simulink library "PECommon"  (Simulink 7.6)
settings: Solver=ode45  StartTime=0.0  StopTime=10.0  RelTol=1e-3
undefined symbols (not defined in the file or in its folder): DiscIntNeverNeededParam, Hydride, Metal, Nickel, Ts, Ts_Discrete
libraries: powerlib x24, simulink x14, PECommon x7, powerlib_extras x7, electricdrivelib x1, simulink_extras x1
(part 1 of 2)
settings Model: Creator=Hu Xaiolei  LastModifiedBy=Mike

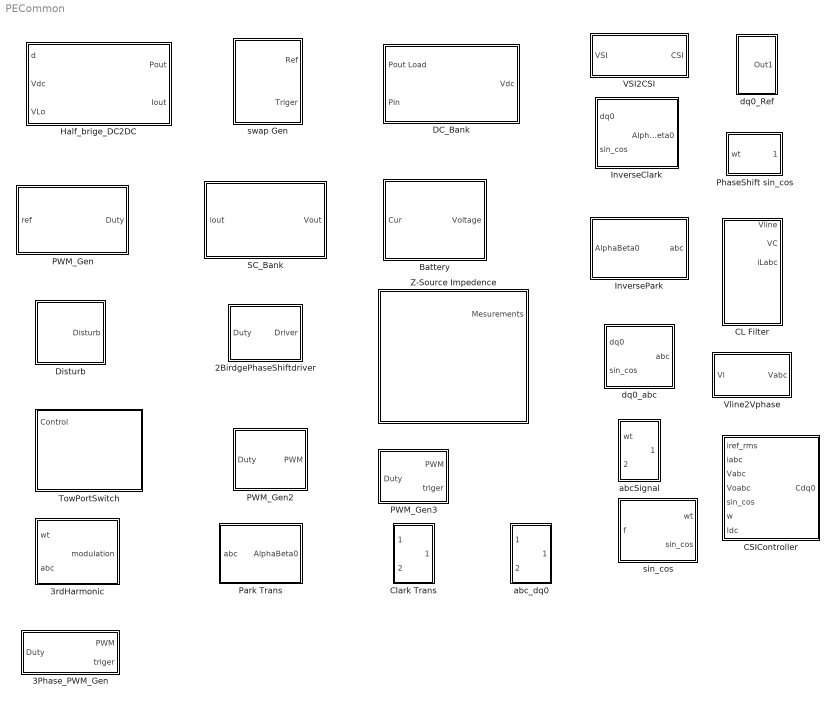
== system PECommon ==
  2BirdgePhaseShiftdriver : Subsystem  mask{fsps=10000}
      mask prompts: fsps "Freq of phase shift control"
      mask init:
      | TsPhaseShift = 1/fsps ;
      mask Display:
      | %plot([2 2 2 3 4 5 6 ],[3 5 5 3 3 5 5])
      | %plot([0 1 2 3 4 5 6 ], [0 0 2 2 0 0 2])
      | plot([0 1],[3 3])
      | plot([0 1],[0 0])
      | plot([1 1],[3 5])
      | plot([1 2],[5 5])
      | plot([1 2],[0 0])
      | plot([2 2],[0 2])
      | plot([2 3],[5 5])
      | plot([2 3],[2 2])
      | plot([3 3],[5 3])
      | plot([3 4],[3 3])
      | plot([3 4],[2 2])
      | plot([4 4],[2 0])
      | plot([4 5],[3 3])
      | plot([4 5],[0 0])
      | plot([5 5],[3 5])
      | plot([5 6],[5 5])
      | plot([5 6],[0 0])
      | plot([6 6],[0 2])
  3Phase_PWM_Gen : Subsystem  mask{Ts_Discrete=1e-6, f_tri=10e3, P_Delay=0}
      mask prompts: Ts_Discrete "Sample Time"; f_tri "Frequency of Sawtooth wave"; P_Delay "Phase Delay"
  3rdHarmonic : Subsystem  mask{SS=Original, ModeCtrl=0}
      mask prompts: SS "Source Selection"; ModeCtrl "Test"
      mask help:
      | 3 phase modulation
      | when Select original, the original A B C sine wave will be present
      | when select 3rd harmonic, 3rd harmonics will be added to A B C to increase
      | the utilization of DC bus.
      mask StyleString: popup(3rd Harmonic|Original),edit
      mask CallbackString:
      | if strcmp(get_param(gcb,'SS'),'Original')
      |     set_param(gcb,'ModeCtrl','0');
      | else
      |     set_param(gcb,'ModeCtrl','1');
      | end|
  Battery : Subsystem  mask{Value=200}
      mask prompts: Value "Battery Normal Voltage"
      mask Display:
      | image(imread('\pic\Battery_Service.jpg'))
      | port_label('input',1,'Current')
      | port_label('output',1,'Voltage')
  CL Filter : Subsystem  mask{L=1000e-6, C=100e-6, R=0.01}
      mask prompts: L "Inductance"; C "Capacitance"
  CSIController : Subsystem  mask{Kc=4.8000, Kp=6.9998, Ki=1.3333e+004, L=1000e-6, C=100e-6}
      mask prompts: Kc "inner loop gain"; Kp "Voltage loop gain"; Ki "Voltage loop integrator gain"; L "Inductance"; C "Capacitance"
  Clark Trans : Subsystem
  DC_Bank : Subsystem  mask{Cdc=0.47, Vdcinit=400}
      mask prompts: Cdc "Capacitance"; Vdcinit "Capacitor initial voltage"
      mask Display:
      | image(imread('\pic\Capacitor.png'))
      | port_label('input',1,'Pout')
      | port_label('input',2,'Pin')
      | port_label('output',1,'Vdc')
  Disturb : Subsystem
      mask Display:
      | image(imread('\pic\Load_Motor.jpg'))
      | port_label('output',1,'Disturb')
  Half_brige_DC2DC : Subsystem  mask{Ls=0.001, imax=1200, imin=-1200, Tsconv=0.0001}
      mask prompts: Ls "Inductance"; imax "Maximum Inductor Current"; imin "Minimum Inductor Current"; Tsconv "Sample Rate"
      mask Display:
      | image(imread('\pic\IGBT.jpg'))
      | disp('Half Brige \n BiD2D')
      | 
      | port_label('input',1,'Duty')
      | port_label('input',2,'Vdc')
      | port_label('input',3,'Vinput')
      | port_label('output',1,'Pout')
      | port_label('output',2,'iL')
  InverseClark : Subsystem
  InversePark : Subsystem
  PWM_Gen : Subsystem  mask{fconvs=1e3}
      mask prompts: fconvs "Switching Freq"
      mask Display:
      | port_label('input',1,'ref')
      | port_label('output',1,'Duty')
      | disp('PWM\nGenerator')
  PWM_Gen2 : Subsystem  mask{Ts_Discrete=Ts_Discrete, f_tri=10e3, P_Delay=0}
      mask prompts: Ts_Discrete "Sample Time"; f_tri "frequency of sawtooth wave"; P_Delay "Arbittary Phase Delay"
  PWM_Gen3 : Subsystem  mask{Ts_Discrete=1e-7, f_tri=10e3, P_Delay=201}
      mask prompts: Ts_Discrete "Sample Time"; f_tri "frequency of sawtooth wave"; P_Delay "Arbittary Phase Delay"
  Park Trans : Subsystem
  PhaseShift sin_cos : Subsystem  mask{Phase=pi/6}
      mask prompts: Phase "Phase Lead"
  SC_Bank : Subsystem  mask{CSC=4.4, Vscinit=254.951}
      mask prompts: CSC "Capacitance"; Vscinit "Initial Voltage"
      mask Display:
      | image(imread('\pic\SuperCapacitor.jpg'))
      | port_label('input',1,'iout')
      | port_label('output',1,'Vout')
  TowPortSwitch : Subsystem
      mask Type: Two Port Switch
      mask Description: When Ctrl is Higher or equal to 1 then, switch port A is connected to port C oherwise, port B is connected to port C
      mask Display:
      | plot([0 10 10 0],[0 0 10 10])
      | plot([1 3 7 9],[5.5 5.5 2 2])
      | plot([1 3],[1.5 1.5])
      | port_label('input',1,'Ctrl')
      | port_label('lconn',1,'A')
      | port_label('lconn',2,'B')
      | port_label('rconn',1,'C')
  VSI2CSI : Subsystem
  Vline2Vphase : Subsystem
  Z-Source Impedence : Subsystem  mask{L1=1e-3, L2=1e-3, C1=1e-6, C2=1e-6}
      mask prompts: L1 "L1 Inductor"; L2 "L2 Inductor"; C1 "C1 Capacitor"; C2 "C2 Capacitor"
      mask Display:
      | image(imread('\pic\ZSource_impedence.png'),'center','on')
      | port_label('Output',1,'Mesurements')
  abcSignal : Subsystem
  abc_dq0 : Subsystem
  dq0_Ref : Subsystem  mask{d=1, q=0, zero=0}
      mask prompts: zero "0"
  dq0_abc : Subsystem
  sin_cos : Subsystem
  swap Gen : Subsystem  mask{fs=10e3}
      mask prompts: fs "swap wave frequency"
      mask Display:
      | port_label('output',1,'Ref')
      | port_label('output',2,'Triger')
      | disp('SWAP\nGen')

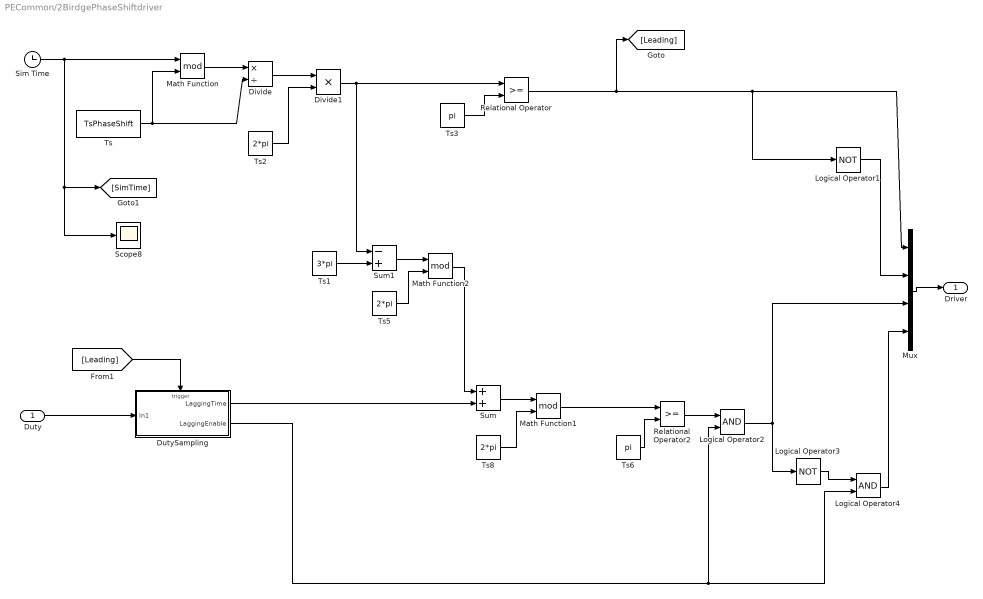
== system PECommon/2BirdgePhaseShiftdriver ==
  Duty : Inport
  Divide : Product  Inputs=*/
  Divide1 : Product  Inputs=**
  DutySampling : Subsystem
  Logical Operator1 : Logic  Operator=NOT  AllPortsSameDT=off  OutDataTypeStr=boolean
  Logical Operator2 : Logic  AllPortsSameDT=off  OutDataTypeStr=boolean
  Logical Operator3 : Logic  Operator=NOT  AllPortsSameDT=off  OutDataTypeStr=boolean
  Logical Operator4 : Logic  AllPortsSameDT=off  OutDataTypeStr=boolean
  Math Function : Math  Operator=mod  SaturateOnIntegerOverflow=on
  Math Function1 : Math  Operator=mod  SaturateOnIntegerOverflow=on
  Math Function2 : Math  Operator=mod  SaturateOnIntegerOverflow=on
  Mux : Mux
  Relational Operator : RelationalOperator  OutDataTypeStr=boolean
  Relational Operator2 : RelationalOperator  OutDataTypeStr=boolean
  Scope8 : Scope
      settings: SaveName=ScopeData8
  Sim Time : Clock
  Sum : Sum
  Sum1 : Sum  Inputs=-+
  Ts : Constant  Value=TsPhaseShift
  Ts1 : Constant  Value=3*pi
  Ts2 : Constant  Value=2*pi
  Ts3 : Constant  Value=pi
  Ts5 : Constant  Value=2*pi
  Ts6 : Constant  Value=pi
  Ts8 : Constant  Value=2*pi
  Driver : Outport
  wires:
  Mux/1 -> Driver/1
  Logical Operator4/1 -> Mux/4
  Logical Operator1/1 -> Mux/2
  Logical Operator3/1 -> Logical Operator4/1
  Sim Time/1 -> Math Function/1, [SimTime], Scope8/1
  Ts/1 -> Math Function/2, Divide/2
  Math Function/1 -> Divide/1
  Divide/1 -> Divide1/1
  Ts2/1 -> Divide1/2
  Divide1/1 -> Relational Operator/1, Sum1/1
  Ts3/1 -> Relational Operator/2
  Relational Operator/1 -> Mux/1, Logical Operator1/1, [Leading]
  Math Function1/1 -> Relational Operator2/1
  Ts6/1 -> Relational Operator2/2
  Ts8/1 -> Math Function1/2
  Sum/1 -> Math Function1/1
  DutySampling/1(LaggingTime) -> Sum/2
  [Leading] -> DutySampling/Trigger
  Ts1/1 -> Sum1/2
  Sum1/1 -> Math Function2/1
  Ts5/1 -> Math Function2/2
  Math Function2/1 -> Sum/1
  Relational Operator2/1 -> Logical Operator2/1
  DutySampling/2(LaggingEnable) -> Logical Operator4/2, Logical Operator2/2
  Logical Operator2/1 -> Mux/3, Logical Operator3/1
  Duty/1 -> DutySampling/1(In1)

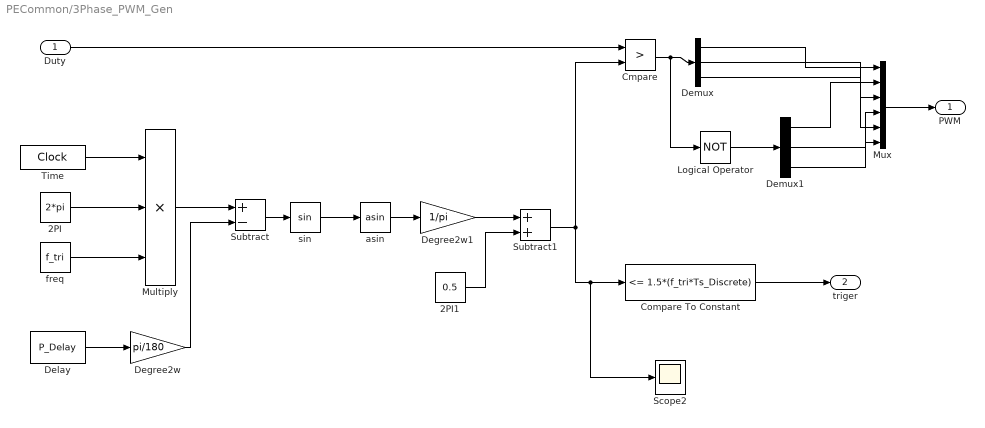
== system PECommon/3Phase_PWM_Gen ==
  Duty : Inport
  2PI : Constant  Value=2*pi
  2PI1 : Constant  Value=0.5
  Cmpare : RelationalOperator  Operator=>  OutDataTypeStr=boolean
  Compare To Constant : simulink/Logic and Bit Operations/Compare To Constant  SystemSampleTime=-1  relop=<=  const=1.5*(f_tri*Ts_Discrete)  LogicOutDataTypeMode=uint8
  Degree2w : Gain  Gain=pi/180
  Degree2w1 : Gain  Gain=1/pi
  Delay : Constant  Value=P_Delay
  Demux : Demux  Outputs=3
  Demux1 : Demux  Outputs=3
  Logical Operator : Logic  Operator=NOT  AllPortsSameDT=off  OutDataTypeStr=boolean
  Multiply : Product  Inputs=***
  Mux : Mux  Inputs=6
  Scope2 : Scope
      settings: SaveName=ScopeData8
  Subtract : Sum  Inputs=+-
  Subtract1 : Sum
  Time : DigitalClock  SampleTime=Ts_Discrete
  asin : Trigonometry  Operator=asin
  freq : Constant  Value=f_tri
  sin : Trigonometry
  PWM : Outport
  triger : Outport  Port=2
  wires:
  Time/1 -> Multiply/1
  2PI/1 -> Multiply/2
  freq/1 -> Multiply/3
  Multiply/1 -> Subtract/1
  Delay/1 -> Degree2w/1
  Degree2w/1 -> Subtract/2
  Subtract/1 -> sin/1
  sin/1 -> asin/1
  asin/1 -> Degree2w1/1
  Degree2w1/1 -> Subtract1/1
  2PI1/1 -> Subtract1/2
  Subtract1/1 -> Cmpare/2, Scope2/1, Compare To Constant/1
  Duty/1 -> Cmpare/1
  Compare To Constant/1 -> triger/1
  Cmpare/1 -> Demux/1, Logical Operator/1
  Logical Operator/1 -> Demux1/1
  Demux/1 -> Mux/1
  Demux1/1 -> Mux/2
  Demux/2 -> Mux/3
  Demux1/2 -> Mux/4
  Demux/3 -> Mux/5
  Demux1/3 -> Mux/6
  Mux/1 -> PWM/1

== system PECommon/3rdHarmonic ==
  wt : Inport
  abc : Inport  Port=2
  Abs : Abs
  Add2 : Sum  Inputs=-+
  Cos6 : Trigonometry  Operator=cos
  Gain1 : Gain  Gain=2/sqrt(3)
  Gain2 : Gain  Gain=3
  Gain7 : Gain  Gain=1/6
  Index Vector : MultiPortSwitch  DataPortOrder=Zero-based contiguous  Inputs=2  zeroidx=on
  ModeCtrl : Constant  Value=ModeCtrl
  Product : Product  RndMeth=Zero
  Saturation1 : Saturate  UpperLimit=1  LowerLimit=-1
  modulation : Outport
  wires:
  Saturation1/1 -> Abs/1, Add2/2, Index Vector/2
  Product/1 -> Add2/1
  Gain7/1 -> Product/2
  Abs/1 -> Product/1
  Gain1/1 -> Index Vector/3
  Cos6/1 -> Gain7/1
  Gain2/1 -> Cos6/1  "3wt"
  wt/1 -> Gain2/1  "wt"
  Add2/1 -> Gain1/1
  Index Vector/1 -> modulation/1
  ModeCtrl/1 -> Index Vector/1
  abc/1 -> Saturation1/1

== system PECommon/Battery ==
  Cur : Inport
  Battery1 : electricdrivelib/Extra Sources/Battery  DialogController=POWERSYS.PowerSysDialog  SystemSampleTime=-1  BatType=Nickel-Metal-Hydride  ShowDetailedParameters=off  NomV=Value  NomQ=1000  SOC=70  PresetModel=on  MaxQ=1076.9231  FullV=235.5932  Dis_rate=200  R=0.002  Normal_OP=961.5385  expZone="[216.9492           200]"  Dis_Char=off  current=[1.5 3]  Units=Ampere-hour  Batt_Tr=30
  CCS : powerlib/Electrical Sources/Controlled Current Source  DialogController=POWERSYS.PowerSysDialog  SystemSampleTime=-1  Initialize=off  Source_Type=DC  Amplitude=0  Phase=0  Frequency=0  Measurements=None
  Terminator : Terminator
  Vm : powerlib/Measurements/Voltage Measurement  DialogController=POWERSYS.PowerSysDialog  SystemSampleTime=-1  PhasorSimulation=off  OutputType=Complex  PSBequivalent=0
  powergui : powerlib/powergui  Priority=1  SystemSampleTime=-1  SimulationMode=Continuous  SampleTime=50e-6  frequency=60  SPID=off  DisableSnubberDevices=off  DisableRonSwitches=off  DisableVfSwitches=off  SwTol=0  Interpol=off  frequencyindice=0  echomessages=off  HookPort=off  DisplayEquations=off  FunctionMessages=off  EnableUseOfTLC=off  x0status=blocks  RestoreLinks=warning  ResistiveCurrentMeasurement=off  Ylog=off  Xlog=on  ShowGrid=off  save=off  variable=ZData  ZoomFFT=off  StartTime=0.0  cycles=1  DisplayStyle=1  FreqAxis=off  MaxFrequency=1000  frequencyindicesteady=1  display=off  methode=off
  Voltage : Outport
  wires:
  Cur/1 -> CCS/1
  Vm/1 -> Voltage/1
  Battery1/1 -> Terminator/1
  connections:
  Vm/LConn2 -- CCS/RConn1 -- Battery1/LConn2
  Vm/LConn1 -- CCS/LConn1 -- Battery1/LConn1

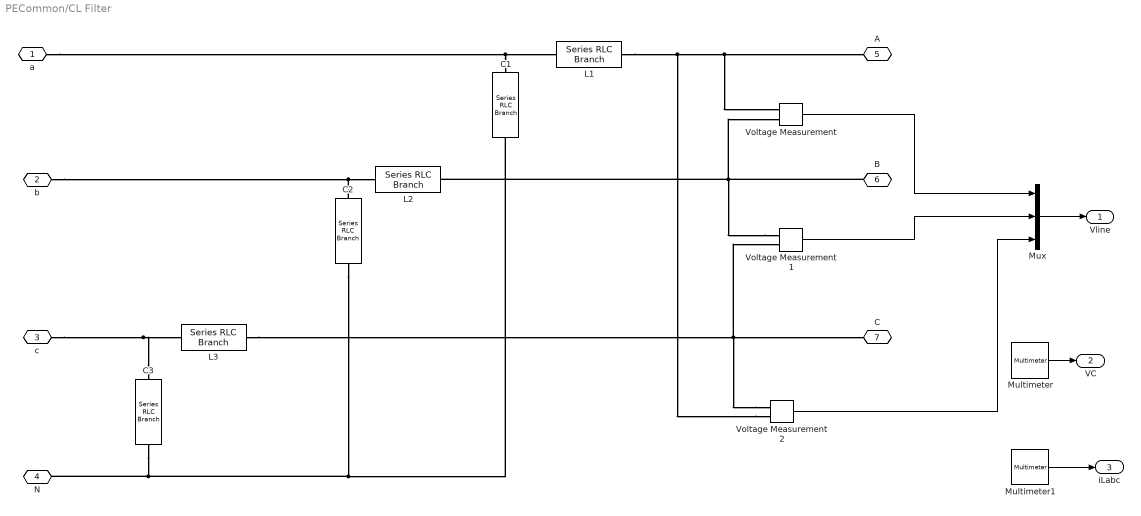
== system PECommon/CL Filter ==
  C1 : powerlib/Elements/Series RLC Branch  DialogController=POWERSYS.PowerSysDialog  PhysicalDomain=powersysdomain  SubClassName=unknown  LeftPortType=p1  RightPortType=p1  LConnTagsString=__new0  RConnTagsString=__new0  BranchType=C  Resistance=1  Inductance=1e-3  SetiL0=off  InitialCurrent=0  Capacitance=C  Setx0=off  InitialVoltage=0  Measurements=Branch voltage and current
  C2 : powerlib/Elements/Series RLC Branch  DialogController=POWERSYS.PowerSysDialog  PhysicalDomain=powersysdomain  SubClassName=unknown  LeftPortType=p1  RightPortType=p1  LConnTagsString=__new0  RConnTagsString=__new0  BranchType=C  Resistance=1  Inductance=1e-3  SetiL0=off  InitialCurrent=0  Capacitance=C  Setx0=off  InitialVoltage=0  Measurements=Branch voltage and current
  C3 : powerlib/Elements/Series RLC Branch  DialogController=POWERSYS.PowerSysDialog  PhysicalDomain=powersysdomain  SubClassName=unknown  LeftPortType=p1  RightPortType=p1  LConnTagsString=__new0  RConnTagsString=__new0  BranchType=C  Resistance=1  Inductance=1e-3  SetiL0=off  InitialCurrent=0  Capacitance=C  Setx0=off  InitialVoltage=0  Measurements=Branch voltage and current
  L1 : powerlib/Elements/Series RLC Branch  DialogController=POWERSYS.PowerSysDialog  PhysicalDomain=powersysdomain  SubClassName=unknown  LeftPortType=p1  RightPortType=p1  LConnTagsString=__new0  RConnTagsString=__new0  BranchType=RL  Resistance=R  Inductance=L  SetiL0=off  InitialCurrent=0  Capacitance=1e-6  Setx0=off  InitialVoltage=0  Measurements=Branch voltage and current
  L2 : powerlib/Elements/Series RLC Branch  DialogController=POWERSYS.PowerSysDialog  PhysicalDomain=powersysdomain  SubClassName=unknown  LeftPortType=p1  RightPortType=p1  LConnTagsString=__new0  RConnTagsString=__new0  BranchType=RL  Resistance=R  Inductance=L  SetiL0=off  InitialCurrent=0  Capacitance=1e-6  Setx0=off  InitialVoltage=0  Measurements=Branch voltage and current
  L3 : powerlib/Elements/Series RLC Branch  DialogController=POWERSYS.PowerSysDialog  PhysicalDomain=powersysdomain  SubClassName=unknown  LeftPortType=p1  RightPortType=p1  LConnTagsString=__new0  RConnTagsString=__new0  BranchType=RL  Resistance=R  Inductance=L  SetiL0=off  InitialCurrent=0  Capacitance=1e-6  Setx0=off  InitialVoltage=0  Measurements=Branch voltage and current
  Multimeter : powerlib/Measurements/Multimeter  SystemSampleTime=-1  PhasorSimulation=off  OutputType=Complex  sel=[1 2 3]  L=12  Gain=[1 1 1]  yselected={'Ub: CL Filter/C1','Ub: CL Filter/C2','Ub: CL Filter/C3'};  PSBOutputType=1  PSBequivalent=0  AxesSetting=[0,0.1,-100,100]  Display=0  SavedBlockNames=-11
  Multimeter1 : powerlib/Measurements/Multimeter  SystemSampleTime=-1  PhasorSimulation=off  OutputType=Complex  sel=[10 11 12]  L=12  Gain=[1 1 1]  yselected={'Ib: CL Filter/L1','Ib: CL Filter/L2','Ib: CL Filter/L3'};  PSBOutputType=1  PSBequivalent=0  AxesSetting=[0,0.1,-100,100]  Display=0  SavedBlockNames=-11
  Mux : Mux  Inputs=3
  Voltage Measurement : powerlib/Measurements/Voltage Measurement  DialogController=POWERSYS.PowerSysDialog  SystemSampleTime=-1  PhasorSimulation=off  OutputType=Complex  PSBequivalent=0
  Voltage Measurement1 : powerlib/Measurements/Voltage Measurement  DialogController=POWERSYS.PowerSysDialog  SystemSampleTime=-1  PhasorSimulation=off  OutputType=Complex  PSBequivalent=0
  Voltage Measurement2 : powerlib/Measurements/Voltage Measurement  DialogController=POWERSYS.PowerSysDialog  SystemSampleTime=-1  PhasorSimulation=off  OutputType=Complex  PSBequivalent=0
  a : PMIOPort  Port=1  Side=Left
  b : PMIOPort  Port=2  Side=Left
  c : PMIOPort  Port=3  Side=Left
  N : PMIOPort  Port=4  Side=Left
  A : PMIOPort  Port=5  Side=Right
  B : PMIOPort  Port=6  Side=Right
  C : PMIOPort  Port=7  Side=Right
  Vline : Outport
  VC : Outport  Port=2
  iLabc : Outport  Port=3
  wires:
  Voltage Measurement2/1 -> Mux/3
  Voltage Measurement1/1 -> Mux/2
  Voltage Measurement/1 -> Mux/1
  Multimeter1/1 -> iLabc/1
  Multimeter/1 -> VC/1
  Mux/1 -> Vline/1
  connections:
  C3/RConn1 -- N/RConn1 -- C2/RConn1 -- C1/RConn1
  Voltage Measurement1/LConn1 -- Voltage Measurement/LConn2 -- L2/RConn1 -- B/RConn1
  Voltage Measurement2/LConn1 -- Voltage Measurement1/LConn2 -- C/RConn1 -- L3/RConn1
  C3/LConn1 -- L3/LConn1 -- c/RConn1
  Voltage Measurement2/LConn2 -- Voltage Measurement/LConn1 -- A/RConn1 -- L1/RConn1
  C1/LConn1 -- L1/LConn1 -- a/RConn1
  b/RConn1 -- L2/LConn1 -- C2/LConn1

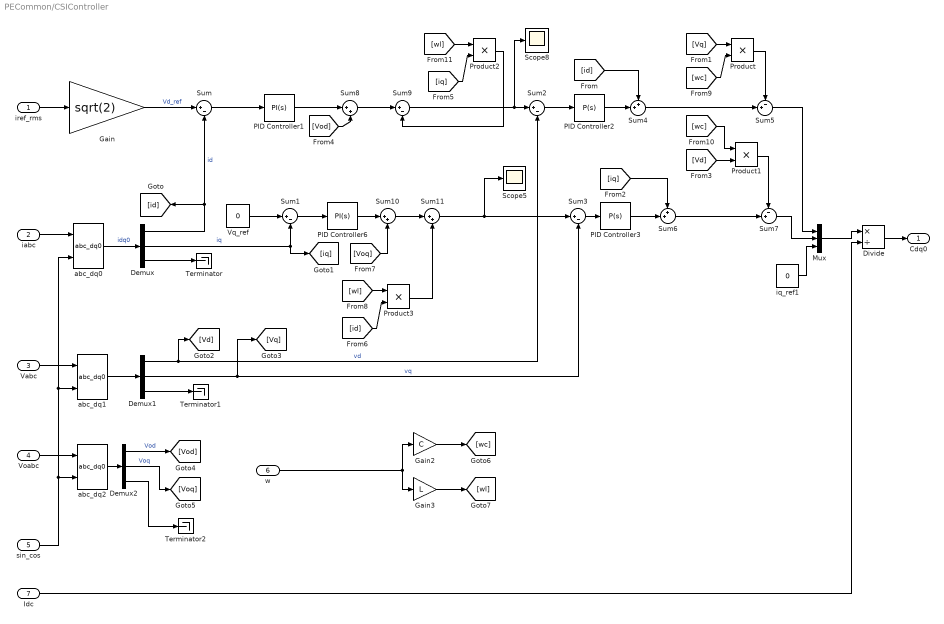
== system PECommon/CSIController ==
  iref_rms : Inport
  iabc : Inport  Port=2
  Vabc : Inport  Port=3
  Voabc : Inport  Port=4
  sin_cos : Inport  Port=5
  w : Inport  Port=6
  Idc : Inport  Port=7
  Demux : Demux  Outputs=3
  Demux1 : Demux  Outputs=3
  Demux2 : Demux  Outputs=3
  Divide : Product  Inputs=*/
  Gain : Gain  Gain=sqrt(2)
  Gain2 : Gain  Gain=C
  Gain3 : Gain  Gain=L
  Mux : Mux  Inputs=3
  PID Controller1 : simulink/Continuous/PID Controller  DialogController=pidpack.PIDConfig.pidDDGCreate  DialogControllerArgs=DataTag0  SystemSampleTime=-1  Controller=PI  TimeDomain=Continuous-time  SampleTime=1  IntegratorMethod=Forward Euler  FilterMethod=Forward Euler  Form=Parallel  P=Kp  I=Ki  D=0  N=100  InitialConditionSource=internal  InitialConditionForIntegrator=0  InitialConditionForFilter=0  ExternalReset=none  LimitOutput=on  UpperSaturationLimit=inf  LowerSaturationLimit=-inf  LinearizeAsGain=off  AntiWindupMode=clamping  Kb=1  TrackingMode=off  Kt=1  PParamMin=[]  PParamMax=[]  IParamMin=[]  IParamMax=[]  DParamMin=[]  DParamMax=[]  NParamMin=[]  NParamMax=[]  KbParamMin=[]  KbParamMax=[]  KtParamMin=[]  KtParamMax=[]  POutMin=[]  POutMax=[]  IOutMin=[]  IOutMax=[]  DOutMin=[]  DOutMax=[]  NOutMin=[]  NOutMax=[]  KbOutMin=[]  KbOutMax=[]  KtOutMin=[]  KtOutMax=[]  IntegratorOutMin=[]  IntegratorOutMax=[]  FilterOutMin=[]  FilterOutMax=[]  SumOutMin=[]  SumOutMax=[]  SumI1OutMin=[]  SumI1OutMax=[]  SumI2OutMin=[]  SumI2OutMax=[]  SumI3OutMin=[]  SumI3OutMax=[]  SumDOutMin=[]  SumDOutMax=[]  SaturationOutMin=[]  SaturationOutMax=[]  IntegratorContinuousStateAttributes=''  IntegratorStateMustResolveToSignalObject=off  IntegratorRTWStateStorageClass=Auto  FilterContinuousStateAttributes=''  FilterStateMustResolveToSignalObject=off  FilterRTWStateStorageClass=Auto
  PID Controller2 : simulink/Continuous/PID Controller  DialogController=pidpack.PIDConfig.pidDDGCreate  DialogControllerArgs=DataTag1  SystemSampleTime=-1  Controller=P  TimeDomain=Continuous-time  SampleTime=1  IntegratorMethod=Forward Euler  FilterMethod=Forward Euler  Form=Ideal  P=Kc  I=0  D=0  N=100  InitialConditionSource=internal  InitialConditionForIntegrator=0  InitialConditionForFilter=0  ExternalReset=none  LimitOutput=off  UpperSaturationLimit=inf  LowerSaturationLimit=-inf  LinearizeAsGain=off  AntiWindupMode=none  Kb=1  TrackingMode=off  Kt=1  PParamMin=[]  PParamMax=[]  IParamMin=[]  IParamMax=[]  DParamMin=[]  DParamMax=[]  NParamMin=[]  NParamMax=[]  KbParamMin=[]  KbParamMax=[]  KtParamMin=[]  KtParamMax=[]  POutMin=[]  POutMax=[]  IOutMin=[]  IOutMax=[]  DOutMin=[]  DOutMax=[]  NOutMin=[]  NOutMax=[]  KbOutMin=[]  KbOutMax=[]  KtOutMin=[]  KtOutMax=[]  IntegratorOutMin=[]  IntegratorOutMax=[]  FilterOutMin=[]  FilterOutMax=[]  SumOutMin=[]  SumOutMax=[]  SumI1OutMin=[]  SumI1OutMax=[]  SumI2OutMin=[]  SumI2OutMax=[]  SumI3OutMin=[]  SumI3OutMax=[]  SumDOutMin=[]  SumDOutMax=[]  SaturationOutMin=[]  SaturationOutMax=[]  IntegratorContinuousStateAttributes=''  IntegratorStateMustResolveToSignalObject=off  IntegratorRTWStateStorageClass=Auto  FilterContinuousStateAttributes=''  FilterStateMustResolveToSignalObject=off  FilterRTWStateStorageClass=Auto
  PID Controller3 : simulink/Continuous/PID Controller  DialogController=pidpack.PIDConfig.pidDDGCreate  DialogControllerArgs=DataTag2  SystemSampleTime=-1  Controller=P  TimeDomain=Continuous-time  SampleTime=1  IntegratorMethod=Forward Euler  FilterMethod=Forward Euler  Form=Ideal  P=Kc  I=0  D=0  N=100  InitialConditionSource=internal  InitialConditionForIntegrator=0  InitialConditionForFilter=0  ExternalReset=none  LimitOutput=off  UpperSaturationLimit=inf  LowerSaturationLimit=-inf  LinearizeAsGain=off  AntiWindupMode=none  Kb=1  TrackingMode=off  Kt=1  PParamMin=[]  PParamMax=[]  IParamMin=[]  IParamMax=[]  DParamMin=[]  DParamMax=[]  NParamMin=[]  NParamMax=[]  KbParamMin=[]  KbParamMax=[]  KtParamMin=[]  KtParamMax=[]  POutMin=[]  POutMax=[]  IOutMin=[]  IOutMax=[]  DOutMin=[]  DOutMax=[]  NOutMin=[]  NOutMax=[]  KbOutMin=[]  KbOutMax=[]  KtOutMin=[]  KtOutMax=[]  IntegratorOutMin=[]  IntegratorOutMax=[]  FilterOutMin=[]  FilterOutMax=[]  SumOutMin=[]  SumOutMax=[]  SumI1OutMin=[]  SumI1OutMax=[]  SumI2OutMin=[]  SumI2OutMax=[]  SumI3OutMin=[]  SumI3OutMax=[]  SumDOutMin=[]  SumDOutMax=[]  SaturationOutMin=[]  SaturationOutMax=[]  IntegratorContinuousStateAttributes=''  IntegratorStateMustResolveToSignalObject=off  IntegratorRTWStateStorageClass=Auto  FilterContinuousStateAttributes=''  FilterStateMustResolveToSignalObject=off  FilterRTWStateStorageClass=Auto
  PID Controller6 : simulink/Continuous/PID Controller  DialogController=pidpack.PIDConfig.pidDDGCreate  DialogControllerArgs=DataTag3  SystemSampleTime=-1  Controller=PI  TimeDomain=Continuous-time  SampleTime=1  IntegratorMethod=Forward Euler  FilterMethod=Forward Euler  Form=Parallel  P=Kp  I=Ki  D=0  N=100  InitialConditionSource=internal  InitialConditionForIntegrator=0  InitialConditionForFilter=0  ExternalReset=none  LimitOutput=on  UpperSaturationLimit=inf  LowerSaturationLimit=-inf  LinearizeAsGain=off  AntiWindupMode=clamping  Kb=1  TrackingMode=off  Kt=1  PParamMin=[]  PParamMax=[]  IParamMin=[]  IParamMax=[]  DParamMin=[]  DParamMax=[]  NParamMin=[]  NParamMax=[]  KbParamMin=[]  KbParamMax=[]  KtParamMin=[]  KtParamMax=[]  POutMin=[]  POutMax=[]  IOutMin=[]  IOutMax=[]  DOutMin=[]  DOutMax=[]  NOutMin=[]  NOutMax=[]  KbOutMin=[]  KbOutMax=[]  KtOutMin=[]  KtOutMax=[]  IntegratorOutMin=[]  IntegratorOutMax=[]  FilterOutMin=[]  FilterOutMax=[]  SumOutMin=[]  SumOutMax=[]  SumI1OutMin=[]  SumI1OutMax=[]  SumI2OutMin=[]  SumI2OutMax=[]  SumI3OutMin=[]  SumI3OutMax=[]  SumDOutMin=[]  SumDOutMax=[]  SaturationOutMin=[]  SaturationOutMax=[]  IntegratorContinuousStateAttributes=''  IntegratorStateMustResolveToSignalObject=off  IntegratorRTWStateStorageClass=Auto  FilterContinuousStateAttributes=''  FilterStateMustResolveToSignalObject=off  FilterRTWStateStorageClass=Auto
  Product{,1..3} (4 alike) : Product  RndMeth=Zero
  Scope5 : Scope
      settings: SaveName=ScopeData7
  Scope8 : Scope
      settings: SaveName=ScopeData14
  Sum{,1..3,9} (5 alike) : Sum  Inputs=|+-
  Sum10 : Sum  Inputs=|++
  Sum11 : Sum  Inputs=|++
  Sum4 : Sum  Inputs=++|
  Sum5 : Sum  Inputs=-+|
  Sum6 : Sum  Inputs=++|
  Sum7 : Sum  Inputs=-+|
  Sum8 : Sum  Inputs=|++
  Terminator : Terminator
  Terminator1 : Terminator
  Terminator2 : Terminator
  Vq_ref : Constant  Value=0
  abc_dq0 : PECommon/abc_dq0  SystemSampleTime=-1
  abc_dq1 : PECommon/abc_dq0  SystemSampleTime=-1
  abc_dq2 : PECommon/abc_dq0  SystemSampleTime=-1
  iq_ref1 : Constant  Value=0
  Cdq0 : Outport
  wires:
  [iq] -> Sum6/1
  Demux2/3 -> Terminator2/1
  Demux1/3 -> Terminator1/1
  Demux/3 -> Terminator/1
  Idc/1 -> Divide/2
  Product1/1 -> Sum7/1
  [wc] -> Product/2
  Product/1 -> Sum5/1
  [id] -> Sum4/1
  Sum5/1 -> Mux/1
  Sum4/1 -> Sum5/2
  PID Controller2/1 -> Sum4/2
  Product3/1 -> Sum11/2
  [wl] -> Product3/1
  [id] -> Product3/2
  Gain3/1 -> [wl]
  Gain2/1 -> [wc]
  w/1 -> Gain3/1, Gain2/1
  [Vod] -> Sum8/2
  Product2/1 -> Sum9/2
  [Voq] -> Sum10/2
  Sum11/1 -> Scope5/1, Sum3/1
  Sum10/1 -> Sum11/1
  PID Controller6/1 -> Sum10/1
  [iq] -> Product2/2
  [wl] -> Product2/1
  Sum9/1 -> Scope8/1, Sum2/1
  Sum8/1 -> Sum9/1
  PID Controller1/1 -> Sum8/1
  Sum7/1 -> Mux/2
  [Vd] -> Product1/2
  Sum6/1 -> Sum7/2
  PID Controller3/1 -> Sum6/2
  [wc] -> Product1/1
  [Vq] -> Product/1
  Divide/1 -> Cdq0/1
  iq_ref1/1 -> Mux/3
  Mux/1 -> Divide/1
  Sum3/1 -> PID Controller3/1
  Sum2/1 -> PID Controller2/1
  Sum1/1 -> PID Controller6/1
  Sum/1 -> PID Controller1/1
  Vq_ref/1 -> Sum1/1
  Demux2/2 -> [Voq]  "Voq"
  Demux2/1 -> [Vod]  "Vod"
  Demux1/2 -> [Vq], Sum3/2  "vq"
  Demux1/1 -> [Vd], Sum2/2  "vd"
  abc_dq2/1 -> Demux2/1
  abc_dq1/1 -> Demux1/1
  sin_cos/1 -> abc_dq1/2, abc_dq0/2, abc_dq2/2
  Voabc/1 -> abc_dq2/1
  Vabc/1 -> abc_dq1/1
  iref_rms/1 -> Gain/1
  Demux/2 -> [iq], Sum1/2  "iq"
  iabc/1 -> abc_dq0/1
  Demux/1 -> [id], Sum/2  "id"
  abc_dq0/1 -> Demux/1  "idq0"
  Gain/1 -> Sum/1  "Vd_ref"

== system PECommon/Clark Trans ==
  AlphaBeta0 : Inport
  sin_cos : Inport  Port=2
  C1 : Constant  Value=0
  C2 : Constant
  Demux1 : Demux  Outputs=2
  Gain : Gain  Gain=-1
  Matrix Concatenate1 : Concatenate  NumInputs=3  Mode=Multidimensional array  ConcatenateDimension=2
  Product : Product  Multiplication=Matrix(*)  RndMeth=Zero
  Vector Concatenate : Concatenate  NumInputs=3  Mode=Vector
  Vector Concatenate1 : Concatenate  NumInputs=3  Mode=Vector
  Vector Concatenate2 : Concatenate  NumInputs=3  Mode=Vector
  dq0 : Outport
  wires:
  AlphaBeta0/1 -> Product/2
  Product/1 -> dq0/1
  sin_cos/1 -> Demux1/1
  Matrix Concatenate1/1 -> Product/1
  Vector Concatenate2/1 -> Matrix Concatenate1/3
  Vector Concatenate1/1 -> Matrix Concatenate1/2
  Vector Concatenate/1 -> Matrix Concatenate1/1
  C2/1 -> Vector Concatenate2/3
  C1/1 -> Vector Concatenate2/2, Vector Concatenate2/1, Vector Concatenate1/3, Vector Concatenate/3
  Gain/1 -> Vector Concatenate/2
  Demux1/2 -> Vector Concatenate1/2, Vector Concatenate/1
  Demux1/1 -> Vector Concatenate1/1, Gain/1

== system PECommon/DC_Bank ==
  Pout Load : Inport
  Pin : Inport  Port=2
  Add : Sum
  Add1 : Sum  Inputs=+-
  Constant : Constant  Value=Vdcinit
  Dc Bank Capacitry : Constant  Value=Cdc
  Divide : Product  Inputs=**
  Divide1 : Product  Inputs=*/
  Integrator : Integrator
  Saturation : Saturate  UpperLimit=1000  LowerLimit=0.1
  Vdc : Outport
  wires:
  Constant/1 -> Add/2
  Integrator/1 -> Add/1
  Add/1 -> Saturation/1
  [Vdc] -> Divide/2
  Dc Bank Capacitry/1 -> Divide/1
  Saturation/1 -> Vdc/1, [Vdc]
  Pin/1 -> Add1/1
  Pout Load/1 -> Add1/2
  Add1/1 -> Divide1/1
  Divide1/1 -> Integrator/1
  Divide/1 -> Divide1/2

== system PECommon/Disturb ==
  Custom : Subsystem  mask{Value=[100,-100,0,50,-50,0], TsCustom=5}
      mask prompts: Value "Value kw"; TsCustom "Step Time"
  Multiport Switch : MultiPortSwitch  zeroidx=off
  Pluse : Subsystem  mask{MaxP=100, MinP=-100, PluseTs=0.1}
      mask prompts: MaxP "Max Power kw"; MinP "Min Power kw"; PluseTs "Duration"
  Scope1 : Scope
  Step : Subsystem  mask{InitP=0, FinalP=100, StepT=0}
      mask prompts: InitP "Initial Power kw"; FinalP "Final Power kw"; StepT "Step Time kw"
  Type : Constant
  Disturb : Outport
  wires:
  Type/1 -> Multiport Switch/1
  Multiport Switch/1 -> Disturb/1
  Step/1(Out1) -> Multiport Switch/2
  Pluse/1(Out1) -> Multiport Switch/3, Scope1/1
  Custom/1(Out1) -> Multiport Switch/4

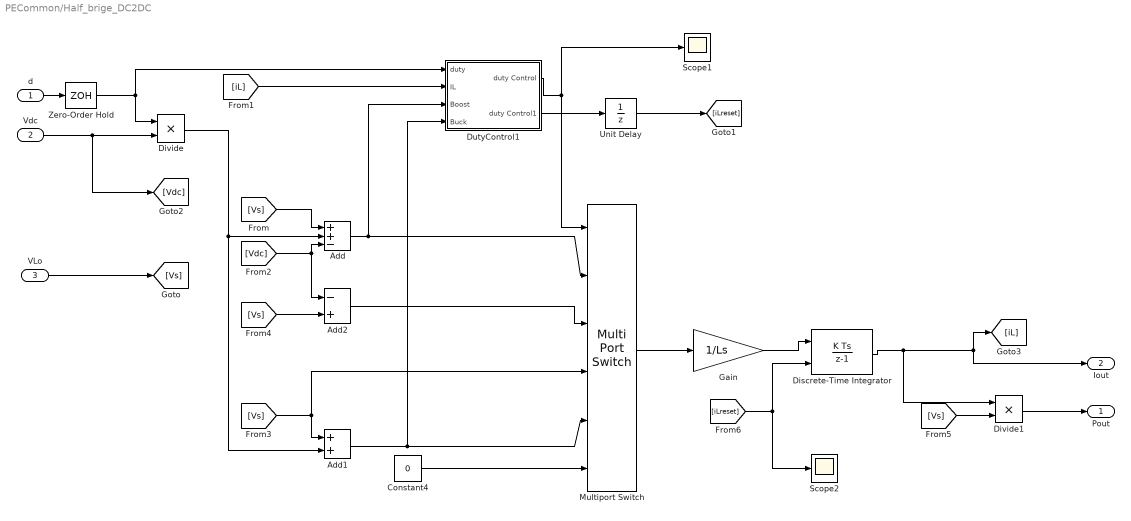
== system PECommon/Half_brige_DC2DC ==
  d : Inport
  Vdc : Inport  Port=2
  VLo : Inport  Port=3
  Add : Sum  Inputs=++-
  Add1 : Sum
  Add2 : Sum  Inputs=-+
  Constant4 : Constant  Value=0
  Discrete-Time Integrator : DiscreteIntegrator  ExternalReset=rising  SampleTime=Tsconv  LimitOutput=on  UpperSaturationLimit=imax  LowerSaturationLimit=imin  ICPrevOutput=DiscIntNeverNeededParam  ICPrevScaledInput=DiscIntNeverNeededParam
  Divide : Product  Inputs=**
  Divide1 : Product  Inputs=**
  DutyControl1 : Subsystem  mask{Tsconv=Tsconv, Ls=Ls}
  Gain : Gain  Gain=1/Ls
  Multiport Switch : MultiPortSwitch  Inputs=5  DiagnosticForDefault=None  zeroidx=off
  Scope1 : Scope
      settings: SaveName=ScopeData11
  Scope2 : Scope
      settings: SaveName=ScopeData12
  Unit Delay : UnitDelay  SampleTime=Tsconv
  Zero-Order Hold : ZeroOrderHold  SampleTime=Tsconv
  Pout : Outport
  Iout : Outport  Port=2
  wires:
  Unit Delay/1 -> [iLreset]
  DutyControl1/2(duty Control1) -> Unit Delay/1
  Zero-Order Hold/1 -> DutyControl1/1(duty), Divide/1
  Discrete-Time Integrator/1 -> Divide1/1, [iL], Iout/1
  [iLreset] -> Discrete-Time Integrator/2, Scope2/1
  [iL] -> DutyControl1/2(IL)
  [Vs] -> Add2/2
  Add2/1 -> Multiport Switch/3
  Add1/1 -> DutyControl1/4(Buck), Multiport Switch/5
  Constant4/1 -> Multiport Switch/6
  DutyControl1/1(duty Control) -> Scope1/1, Multiport Switch/1
  Multiport Switch/1 -> Gain/1
  Add/1 -> DutyControl1/3(Boost), Multiport Switch/2
  d/1 -> Zero-Order Hold/1
  Divide1/1 -> Pout/1
  [Vs] -> Divide1/2
  [Vs] -> Multiport Switch/4, Add1/1
  [Vdc] -> Add2/1, Add/3
  [Vs] -> Add/1
  Divide/1 -> Add/2, Add1/2
  VLo/1 -> [Vs]
  Gain/1 -> Discrete-Time Integrator/1
  Vdc/1 -> [Vdc], Divide/2

== system PECommon/InverseClark ==
  dq0 : Inport
  sin_cos : Inport  Port=2
  C1 : Constant
  C2 : Constant  Value=0
  Demux : Demux  Outputs=2
  Gain : Gain  Gain=-1
  Matrix Concatenate1 : Concatenate  NumInputs=3  Mode=Multidimensional array  ConcatenateDimension=2
  Product : Product  Multiplication=Matrix(*)  RndMeth=Zero
  Vector Concatenate : Concatenate  NumInputs=3  Mode=Vector
  Vector Concatenate1 : Concatenate  NumInputs=3  Mode=Vector
  Vector Concatenate2 : Concatenate  NumInputs=3  Mode=Vector
  AlphaBeta0 : Outport
  wires:
  dq0/1 -> Product/2
  Product/1 -> AlphaBeta0/1
  sin_cos/1 -> Demux/1
  Gain/1 -> Vector Concatenate1/1
  Demux/2 -> Vector Concatenate1/2, Vector Concatenate/1
  Demux/1 -> Vector Concatenate/2, Gain/1  "sin"
  Matrix Concatenate1/1 -> Product/1
  Vector Concatenate2/1 -> Matrix Concatenate1/3
  Vector Concatenate1/1 -> Matrix Concatenate1/2
  Vector Concatenate/1 -> Matrix Concatenate1/1
  C1/1 -> Vector Concatenate2/3
  C2/1 -> Vector Concatenate2/2, Vector Concatenate2/1, Vector Concatenate1/3, Vector Concatenate/3

== system PECommon/InversePark ==
  AlphaBeta0 : Inport
  Constant : Constant  Value=[1 0 1; -1/2 sqrt(3)/2 1;-1/2 -sqrt(3)/2 1]  VectorParams1D=off
  Product1 : Product  Multiplication=Matrix(*)  RndMeth=Zero
  abc : Outport
  wires:
  AlphaBeta0/1 -> Product1/2
  Product1/1 -> abc/1
  Constant/1 -> Product1/1

== system PECommon/PWM_Gen ==
  ref : Inport
  Add : Sum
  Constant1 : Constant  Value=-1
  Demux3 : Demux  Outputs=2
  Gain : Gain  Gain=2
  PWM Generator : powerlib_extras/Control  Blocks/PWM Generator  DialogController=POWERSYS.PowerSysDialog  SystemSampleTime=-1  GeneratorMode="1-arm  bridge (2 pulses)"  Fc=fconvs  Internal=off  mIndex=0  Freq=0  Phase=0
  Terminator : Terminator
  Duty : Outport
  wires:
  PWM Generator/1 -> Demux3/1
  Gain/1 -> Add/1
  Constant1/1 -> Add/2
  Demux3/1 -> Duty/1
  ref/1 -> Gain/1
  Demux3/2 -> Terminator/1
  Add/1 -> PWM Generator/1

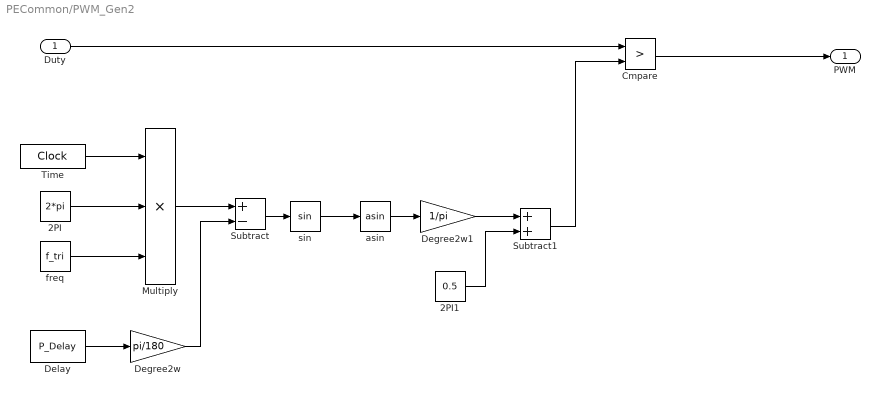
== system PECommon/PWM_Gen2 ==
  Duty : Inport
  2PI : Constant  Value=2*pi
  2PI1 : Constant  Value=0.5
  Cmpare : RelationalOperator  Operator=>  OutDataTypeStr=boolean
  Degree2w : Gain  Gain=pi/180
  Degree2w1 : Gain  Gain=1/pi
  Delay : Constant  Value=P_Delay
  Multiply : Product  Inputs=***
  Subtract : Sum  Inputs=+-
  Subtract1 : Sum
  Time : DigitalClock  SampleTime=Ts_Discrete
  asin : Trigonometry  Operator=asin
  freq : Constant  Value=f_tri
  sin : Trigonometry
  PWM : Outport
  wires:
  Cmpare/1 -> PWM/1
  Duty/1 -> Cmpare/1
  Subtract1/1 -> Cmpare/2
  2PI1/1 -> Subtract1/2
  Degree2w1/1 -> Subtract1/1
  asin/1 -> Degree2w1/1
  sin/1 -> asin/1
  Subtract/1 -> sin/1
  Degree2w/1 -> Subtract/2
  Delay/1 -> Degree2w/1
  Multiply/1 -> Subtract/1
  freq/1 -> Multiply/3
  2PI/1 -> Multiply/2
  Time/1 -> Multiply/1

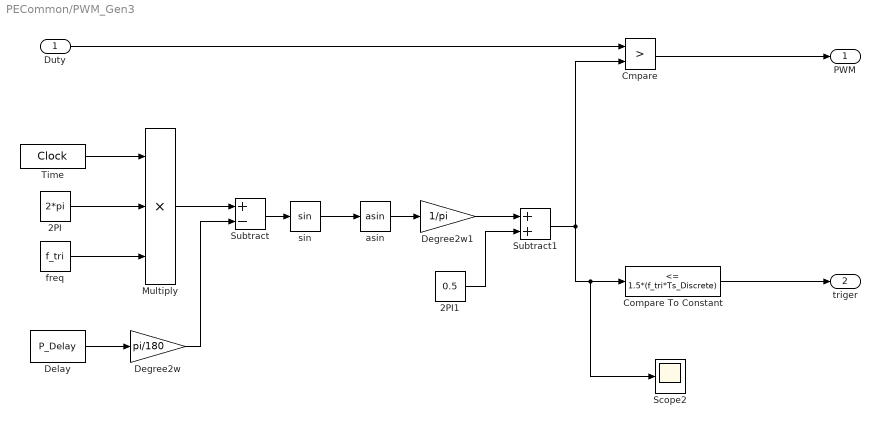
== system PECommon/PWM_Gen3 ==
  Duty : Inport
  2PI : Constant  Value=2*pi
  2PI1 : Constant  Value=0.5
  Cmpare : RelationalOperator  Operator=>  OutDataTypeStr=boolean
  Compare To Constant : simulink/Logic and Bit Operations/Compare To Constant  SystemSampleTime=-1  relop=<=  const=1.5*(f_tri*Ts_Discrete)  LogicOutDataTypeMode=uint8
  Degree2w : Gain  Gain=pi/180
  Degree2w1 : Gain  Gain=1/pi
  Delay : Constant  Value=P_Delay
  Multiply : Product  Inputs=***
  Scope2 : Scope
      settings: SaveName=ScopeData12
  Subtract : Sum  Inputs=+-
  Subtract1 : Sum
  Time : DigitalClock  SampleTime=Ts_Discrete
  asin : Trigonometry  Operator=asin
  freq : Constant  Value=f_tri
  sin : Trigonometry
  PWM : Outport
  triger : Outport  Port=2
  wires:
  Compare To Constant/1 -> triger/1
  Cmpare/1 -> PWM/1
  Duty/1 -> Cmpare/1
  Subtract1/1 -> Compare To Constant/1, Scope2/1, Cmpare/2
  2PI1/1 -> Subtract1/2
  Degree2w1/1 -> Subtract1/1
  asin/1 -> Degree2w1/1
  sin/1 -> asin/1
  Subtract/1 -> sin/1
  Degree2w/1 -> Subtract/2
  Delay/1 -> Degree2w/1
  Multiply/1 -> Subtract/1
  freq/1 -> Multiply/3
  2PI/1 -> Multiply/2
  Time/1 -> Multiply/1

== system PECommon/Park Trans ==
  abc : Inport
  Constant : Constant  Value=[1 -1/2 -1/2;0 sqrt(3)/2 -sqrt(3)/2;1/2 1/2 1/2]  VectorParams1D=off
  Constant1 : Constant  Value=2/3  VectorParams1D=off
  Product : Product  RndMeth=Zero
  Product1 : Product  Multiplication=Matrix(*)  RndMeth=Zero
  AlphaBeta0 : Outport
  wires:
  Product1/1 -> AlphaBeta0/1
  abc/1 -> Product/1
  Constant/1 -> Product1/1
  Product/1 -> Product1/2
  Constant1/1 -> Product/2

== system PECommon/PhaseShift sin_cos ==
  wt : Inport
  Constant1 : Constant  Value=Phase
  Mux : Mux  Inputs=2
  Sum : Sum  Inputs=|++
  Trigonometric Function : Trigonometry
  Trigonometric Function1 : Trigonometry  Operator=cos
  Sin_cos : Outport
  wires:
  Mux/1 -> Sin_cos/1
  wt/1 -> Sum/1
  Trigonometric Function1/1 -> Mux/2
  Trigonometric Function/1 -> Mux/1
  Sum/1 -> Trigonometric Function1/1, Trigonometric Function/1
  Constant1/1 -> Sum/2

== system PECommon/SC_Bank ==
  iout : Inport
  Add : Sum  Inputs=-+
  Constant3 : Constant  Value=1/CSC
  Constant4 : Constant  Value=Vscinit
  Divide : Product  Inputs=**
  Integrator : Integrator
  Saturation : Saturate  UpperLimit=1000  LowerLimit=0.1
  Vout : Outport
  wires:
  iout/1 -> Divide/1
  Constant3/1 -> Divide/2
  Divide/1 -> Integrator/1
  Integrator/1 -> Add/1
  Constant4/1 -> Add/2
  Add/1 -> Saturation/1
  Saturation/1 -> Vout/1

== system PECommon/TowPortSwitch ==
  Control : Inport
  Compare To Constant : simulink/Logic and Bit Operations/Compare To Constant  SystemSampleTime=-1  relop=>=  const=1.0  LogicOutDataTypeMode=boolean
  Ideal Switch : powerlib/Power Electronics/Ideal Switch  DialogController=POWERSYS.PowerSysDialog  SystemSampleTime=-1  Ron=0.001  Lon=0  IC=1  Rs=1e5  Cs=inf  Measurements=on
  Ideal Switch1 : powerlib/Power Electronics/Ideal Switch  DialogController=POWERSYS.PowerSysDialog  SystemSampleTime=-1  Ron=0.001  Lon=0  IC=0  Rs=1e5  Cs=inf  Measurements=on
  Logical Operator : Logic  Operator=NOT  AllPortsSameDT=off  OutDataTypeStr=boolean
  Conn1 : PMIOPort  Port=1  Side=Left
  Conn2 : PMIOPort  Port=2  Side=Left
  Comon : PMIOPort  Port=3  Side=Right
  wires:
  Logical Operator/1 -> Ideal Switch1/1
  Compare To Constant/1 -> Ideal Switch/1, Logical Operator/1
  Control/1 -> Compare To Constant/1
  connections:
  Comon/RConn1 -- Ideal Switch1/RConn1 -- Ideal Switch/RConn1
  Conn2/RConn1 -- Ideal Switch1/LConn1
  Conn1/RConn1 -- Ideal Switch/LConn1

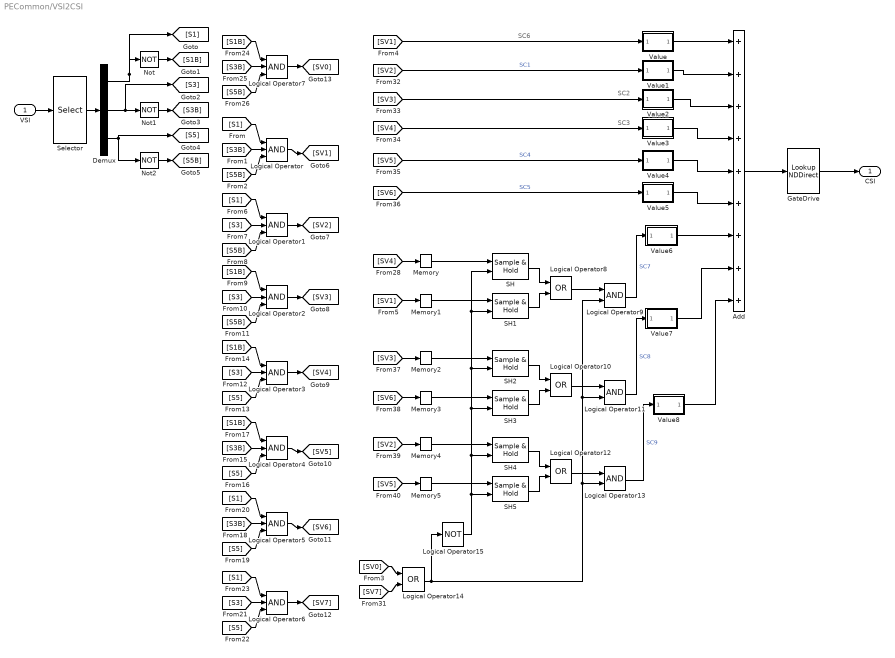
== system PECommon/VSI2CSI ==
  note: SC3
  note: SC2
  note: SC6
  VSI : Inport
  Add : Sum  Inputs=+++++++++
  Demux : Demux  Outputs=3
  GateDrive : LookupNDDirect  InputsSelectThisObjectFromTable=Column  Table=reshape([0,0,0,0,0,0,1,0,0,0,0,1,0,0,1,0,0,1,0,1,1,0,0,0,0,1,0,0,1,0,0,0,0,1,1,0,1,0,0,1,0,0,1,1,0,0,0,0,0,0,1,1,0,0,0,0,0,0,1,1],6,10)
  Logical Operator{,1..7} (8 alike) : Logic  Inputs=3  AllPortsSameDT=off  OutDataTypeStr=boolean
  Logical Operator{8,10,12,14} (4 alike) : Logic  Operator=OR  AllPortsSameDT=off  OutDataTypeStr=boolean
  Logical Operator11 : Logic  AllPortsSameDT=off  OutDataTypeStr=boolean
  Logical Operator13 : Logic  AllPortsSameDT=off  OutDataTypeStr=boolean
  Logical Operator15 : Logic  Operator=NOT  AllPortsSameDT=off  OutDataTypeStr=boolean
  Logical Operator9 : Logic  AllPortsSameDT=off  OutDataTypeStr=boolean
  Memory{,1..5} (6 alike) : Memory
  Not : Logic  Operator=NOT  AllPortsSameDT=off  OutDataTypeStr=boolean
  Not1 : Logic  Operator=NOT  AllPortsSameDT=off  OutDataTypeStr=boolean
  Not2 : Logic  Operator=NOT  AllPortsSameDT=off  OutDataTypeStr=boolean
  SH{,1..5} (6 alike) : powerlib_extras/Control  Blocks/Sample & Hold  DialogController=POWERSYS.PowerSysDialog  SystemSampleTime=-1  ic=0
  Selector : Selector  InputPortWidth=6  IndexOptions=Index vector (dialog)  Indices=[1 3 5]  OutputSizes=1
  Value : Subsystem  mask{Value=6}
  Value1 : Subsystem  mask{Value=1}
  Value2 : Subsystem  mask{Value=2}
  Value3 : Subsystem  mask{Value=3}
  Value4 : Subsystem  mask{Value=4}
  Value5 : Subsystem  mask{Value=5}
  Value6 : Subsystem  mask{Value=7}
  Value7 : Subsystem  mask{Value=8}
  Value8 : Subsystem  mask{Value=9}
  CSI : Outport
  wires:
  Value8/1(Out1) -> Add/9
  Value7/1(Out1) -> Add/8
  Value6/1(Out1) -> Add/7
  Value5/1(Out1) -> Add/6
  Value4/1(Out1) -> Add/5
  Value3/1(Out1) -> Add/4
  Value2/1(Out1) -> Add/3
  Value1/1(Out1) -> Add/2
  Value/1(Out1) -> Add/1
  GateDrive/1 -> CSI/1
  Add/1 -> GateDrive/1
  Logical Operator15/1 -> SH5/2, SH4/2, SH3/2, SH2/2, SH1/2, SH/2
  Logical Operator14/1 -> Logical Operator15/1, Logical Operator13/2, Logical Operator11/2, Logical Operator9/2
  [SV7] -> Logical Operator14/2
  [SV0] -> Logical Operator14/1
  Logical Operator13/1 -> Value8/1(In1)  "SC9"
  Logical Operator12/1 -> Logical Operator13/1
  SH5/1 -> Logical Operator12/2
  SH4/1 -> Logical Operator12/1
  Memory5/1 -> SH5/1
  Memory4/1 -> SH4/1
  [SV5] -> Memory5/1
  [SV2] -> Memory4/1
  Logical Operator11/1 -> Value7/1(In1)  "SC8"
  Logical Operator10/1 -> Logical Operator11/1
  SH3/1 -> Logical Operator10/2
  SH2/1 -> Logical Operator10/1
  Memory3/1 -> SH3/1
  Memory2/1 -> SH2/1
  [SV6] -> Memory3/1
  [SV3] -> Memory2/1
  Logical Operator9/1 -> Value6/1(In1)  "SC7"
  Logical Operator8/1 -> Logical Operator9/1
  SH1/1 -> Logical Operator8/2
  SH/1 -> Logical Operator8/1
  Memory1/1 -> SH1/1
  Memory/1 -> SH/1
  [SV1] -> Memory1/1
  [SV4] -> Memory/1
  [SV6] -> Value5/1(In1)  "SC5"
  [SV5] -> Value4/1(In1)  "SC4"
  [SV4] -> Value3/1(In1)
  [SV3] -> Value2/1(In1)
  [SV2] -> Value1/1(In1)  "SC1"
  [SV1] -> Value/1(In1)
  Logical Operator7/1 -> [SV0]
  [S5B] -> Logical Operator7/3
  [S3B] -> Logical Operator7/2
  [S1B] -> Logical Operator7/1
  Logical Operator6/1 -> [SV7]
  [S5] -> Logical Operator6/3
  [S3] -> Logical Operator6/2
  [S1] -> Logical Operator6/1
  Logical Operator5/1 -> [SV6]
  [S5] -> Logical Operator5/3
  [S3B] -> Logical Operator5/2
  [S1] -> Logical Operator5/1
  Logical Operator4/1 -> [SV5]
  [S5] -> Logical Operator4/3
  [S3B] -> Logical Operator4/2
  [S1B] -> Logical Operator4/1
  Logical Operator3/1 -> [SV4]
  [S5] -> Logical Operator3/3
  [S3] -> Logical Operator3/2
  [S1B] -> Logical Operator3/1
  Logical Operator2/1 -> [SV3]
  [S5B] -> Logical Operator2/3
  [S3] -> Logical Operator2/2
  [S1B] -> Logical Operator2/1
  Logical Operator1/1 -> [SV2]
  [S5B] -> Logical Operator1/3
  [S3] -> Logical Operator1/2
  [S1] -> Logical Operator1/1
  Logical Operator/1 -> [SV1]
  [S5B] -> Logical Operator/3
  [S3B] -> Logical Operator/2
  [S1] -> Logical Operator/1
  Not2/1 -> [S5B]
  Not1/1 -> [S3B]
  Not/1 -> [S1B]
  Demux/3 -> [S5], Not2/1
  Demux/2 -> [S3], Not1/1
  Demux/1 -> [S1], Not/1
  Selector/1 -> Demux/1
  VSI/1 -> Selector/1

== system PECommon/Vline2Vphase ==
  Vl : Inport
  Demux : Demux  Outputs=3
  Gain : Gain  Gain=2/3
  Gain1 : Gain  Gain=1/3
  Gain2 : Gain  Gain=-1/3
  Gain3 : Gain  Gain=1/3
  Mux : Mux  Inputs=3
  Subtract : Sum
  Subtract1 : Sum
  Subtract2 : Sum  Inputs=--
  Terminator : Terminator
  Vabc : Outport
  wires:
  Mux/1 -> Vabc/1
  Subtract2/1 -> Mux/3
  Subtract1/1 -> Mux/2, Subtract2/2
  Subtract/1 -> Mux/1, Subtract2/1
  Demux/2 -> Gain3/1, Gain1/1
  Demux/1 -> Gain2/1, Gain/1
  Gain3/1 -> Subtract1/2
  Gain2/1 -> Subtract1/1
  Gain1/1 -> Subtract/2
  Gain/1 -> Subtract/1
  Demux/3 -> Terminator/1
  Vl/1 -> Demux/1

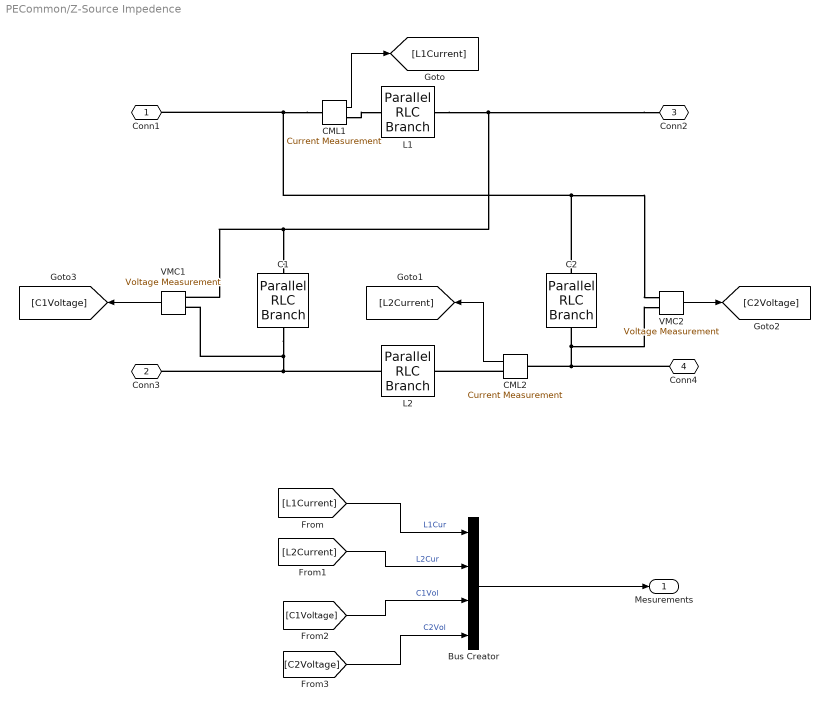
== system PECommon/Z-Source Impedence ==
  Bus Creator : BusCreator
  C1 : powerlib/Elements/Parallel RLC Branch  DialogController=POWERSYS.PowerSysDialog  PhysicalDomain=powersysdomain  SubClassName=unknown  LeftPortType=p1  RightPortType=p1  LConnTagsString=a  RConnTagsString=__new0  BranchType=C  Resistance=1  Inductance=1e-3  SetiL0=off  InitialCurrent=0  Capacitance=C1  Setx0=off  InitialVoltage=0  Measurements=None
  C2 : powerlib/Elements/Parallel RLC Branch  DialogController=POWERSYS.PowerSysDialog  PhysicalDomain=powersysdomain  SubClassName=unknown  LeftPortType=p1  RightPortType=p1  LConnTagsString=a  RConnTagsString=__new0  BranchType=C  Resistance=1  Inductance=1e-3  SetiL0=off  InitialCurrent=0  Capacitance=C2  Setx0=off  InitialVoltage=0  Measurements=None
  CML1 : powerlib/Measurements/Current Measurement  DialogController=POWERSYS.PowerSysDialog  SystemSampleTime=-1  PhasorSimulation=off  OutputType=Complex  PSBequivalent=0
  CML2 : powerlib/Measurements/Current Measurement  DialogController=POWERSYS.PowerSysDialog  SystemSampleTime=-1  PhasorSimulation=off  OutputType=Complex  PSBequivalent=0
  L1 : powerlib/Elements/Parallel RLC Branch  DialogController=POWERSYS.PowerSysDialog  PhysicalDomain=powersysdomain  SubClassName=unknown  LeftPortType=p1  RightPortType=p1  LConnTagsString=a  RConnTagsString=__new0  BranchType=L  Resistance=1  Inductance=L1  SetiL0=off  InitialCurrent=0  Capacitance=1e-6  Setx0=off  InitialVoltage=0  Measurements=None
  L2 : powerlib/Elements/Parallel RLC Branch  DialogController=POWERSYS.PowerSysDialog  PhysicalDomain=powersysdomain  SubClassName=unknown  LeftPortType=p1  RightPortType=p1  LConnTagsString=a  RConnTagsString=__new0  BranchType=L  Resistance=1  Inductance=L2  SetiL0=off  InitialCurrent=0  Capacitance=1e-6  Setx0=off  InitialVoltage=0  Measurements=None
  VMC1 : powerlib/Measurements/Voltage Measurement  DialogController=POWERSYS.PowerSysDialog  SystemSampleTime=-1  PhasorSimulation=off  OutputType=Complex  PSBequivalent=0
  VMC2 : powerlib/Measurements/Voltage Measurement  DialogController=POWERSYS.PowerSysDialog  SystemSampleTime=-1  PhasorSimulation=off  OutputType=Complex  PSBequivalent=0
  Conn1 : PMIOPort  Port=1  Side=Left
  Conn3 : PMIOPort  Port=2  Side=Left
  Conn2 : PMIOPort  Port=3  Side=Right
  Conn4 : PMIOPort  Port=4  Side=Right
  Mesurements : Outport
      settings: VarSizeSig=Yes
  wires:
  CML1/1 -> [L1Current]
  CML2/1 -> [L2Current]
  VMC2/1 -> [C2Voltage]
  VMC1/1 -> [C1Voltage]
  Bus Creator/1 -> Mesurements/1
  [L1Current] -> Bus Creator/1  "L1Cur"
  [L2Current] -> Bus Creator/2  "L2Cur"
  [C2Voltage] -> Bus Creator/4  "C2Vol"
  [C1Voltage] -> Bus Creator/3  "C1Vol"
  connections:
  CML2/LConn1 -- C2/RConn1 -- VMC2/LConn2 -- Conn4/RConn1
  L2/LConn1 -- C1/RConn1 -- VMC1/LConn2 -- Conn3/RConn1
  CML1/LConn1 -- C2/LConn1 -- VMC2/LConn1 -- Conn1/RConn1
  Conn2/RConn1 -- C1/LConn1 -- VMC1/LConn1 -- L1/RConn1
  CML1/RConn1 -- L1/LConn1
  CML2/RConn1 -- L2/RConn1

== system PECommon/abcSignal ==
  wt : Inport
  Amp : Inport  Port=2
  Constant : Constant  Value=-2*pi/3
  Constant1 : Constant  Value=2*pi/3
  Mux : Mux  Inputs=3
  Product : Product  RndMeth=Zero
  Sum : Sum  Inputs=|++
  Sum1 : Sum  Inputs=|++
  Trigonometric Function : Trigonometry  Operator=cos
  abc : Outport
  wires:
  Amp/1 -> Product/2
  Product/1 -> abc/1
  wt/1 -> Sum1/1, Sum/1, Mux/1
  Trigonometric Function/1 -> Product/1
  Mux/1 -> Trigonometric Function/1
  Sum1/1 -> Mux/3
  Constant1/1 -> Sum1/2
  Sum/1 -> Mux/2
  Constant/1 -> Sum/2

== system PECommon/abc_dq0 ==
  abc : Inport
  sin_cos : Inport  Port=2
  Clark Trans : PECommon/Clark Trans  SystemSampleTime=-1
  Park Trans : PECommon/Park Trans  SystemSampleTime=-1
  dq0 : Outport
  wires:
  sin_cos/1 -> Clark Trans/2
  Clark Trans/1 -> dq0/1
  abc/1 -> Park Trans/1
  Park Trans/1 -> Clark Trans/1

== system PECommon/dq0_Ref ==
  Constant2 : Constant  Value=d
  Constant3 : Constant  Value=q
  Constant4 : Constant  Value=zero
  Mux1 : Mux  Inputs=3
  Out1 : Outport
  wires:
  Mux1/1 -> Out1/1
  Constant4/1 -> Mux1/3
  Constant3/1 -> Mux1/2
  Constant2/1 -> Mux1/1

== system PECommon/dq0_abc ==
  dq0 : Inport
  sin_cos : Inport  Port=2
  InverseClark1 : PECommon/InverseClark  SystemSampleTime=-1
  InversePark1 : PECommon/InversePark  SystemSampleTime=-1
  abc : Outport
  wires:
  sin_cos/1 -> InverseClark1/2
  InversePark1/1 -> abc/1
  dq0/1 -> InverseClark1/1
  InverseClark1/1 -> InversePark1/1

== system PECommon/sin_cos ==
  f : Inport
  Clock : Clock
      settings: Decimation=10
  Constant1 : Constant  Value=2*pi
  Cos1 : Trigonometry  Operator=cos
  Cos7 : Trigonometry
  Mux3 : Mux  Inputs=2
  Product : Product  RndMeth=Zero
  Product1 : Product  RndMeth=Zero
  wt : Outport
  sin_cos : Outport  Port=2
  wires:
  Cos1/1 -> Mux3/2
  Cos7/1 -> Mux3/1
  Mux3/1 -> sin_cos/1
  f/1 -> Product/1
  Product1/1 -> Cos1/1, Cos7/1, wt/1
  Constant1/1 -> Product/2
  Product/1 -> Product1/2
  Clock/1 -> Product1/1

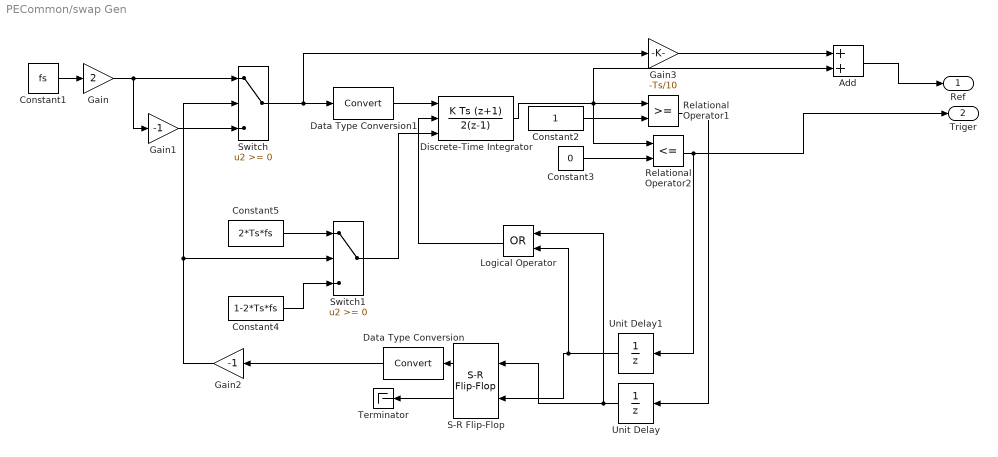
== system PECommon/swap Gen ==
  Add : Sum
  Constant1 : Constant  Value=fs
  Constant2 : Constant
  Constant3 : Constant  Value=0
  Constant4 : Constant  Value=1-2*Ts*fs
  Constant5 : Constant  Value=2*Ts*fs
  Data Type Conversion : DataTypeConversion  SaturateOnIntegerOverflow=on  RndMeth=Zero
  Data Type Conversion1 : DataTypeConversion  SaturateOnIntegerOverflow=on  RndMeth=Zero
  Discrete-Time Integrator : DiscreteIntegrator  IntegratorMethod=Integration: Trapezoidal  ExternalReset=rising  InitialConditionSource=external  InitialCondition=2*Ts*fs  SampleTime=Ts  UpperSaturationLimit=1.5  LowerSaturationLimit=-1.5  ICPrevOutput=DiscIntNeverNeededParam  ICPrevScaledInput=DiscIntNeverNeededParam
  Gain : Gain  Gain=2  SampleTime=Ts
  Gain1 : Gain  Gain=-1  SampleTime=Ts
  Gain2 : Gain  Gain=-1  SampleTime=Ts
  Gain3 : Gain  Gain=-Ts/10  SampleTime=Ts
  Logical Operator : Logic  Operator=OR  AllPortsSameDT=off  OutDataTypeStr=boolean
  Relational Operator1 : RelationalOperator  SampleTime=Ts
  Relational Operator2 : RelationalOperator  Operator=<=  SampleTime=Ts
  S-R Flip-Flop : simulink_extras/Flip Flops/S-R Flip-Flop  SystemSampleTime=-1  initial_condition=0
  Switch : Switch  SampleTime=Ts
  Switch1 : Switch  SampleTime=Ts
  Terminator : Terminator
  Unit Delay : UnitDelay  SampleTime=Ts
  Unit Delay1 : UnitDelay  SampleTime=Ts
  Ref : Outport
  Triger : Outport  Port=2
  wires:
  Relational Operator1/1 -> Unit Delay/1
  Constant2/1 -> Relational Operator1/2
  Discrete-Time Integrator/1 -> Relational Operator1/1, Relational Operator2/1, Add/2
  Constant1/1 -> Gain/1
  Gain/1 -> Switch/1, Gain1/1
  Gain1/1 -> Switch/3
  Switch/1 -> Data Type Conversion1/1, Gain3/1
  Constant3/1 -> Relational Operator2/2
  Relational Operator2/1 -> Unit Delay1/1, Triger/1
  Data Type Conversion/1 -> Gain2/1
  S-R Flip-Flop/1 -> Data Type Conversion/1
  Gain2/1 -> Switch/2, Switch1/2
  Unit Delay/1 -> S-R Flip-Flop/1, Logical Operator/1
  Unit Delay1/1 -> S-R Flip-Flop/2, Logical Operator/2
  Data Type Conversion1/1 -> Discrete-Time Integrator/1
  Switch1/1 -> Discrete-Time Integrator/3
  Constant5/1 -> Switch1/1
  Constant4/1 -> Switch1/3
  Logical Operator/1 -> Discrete-Time Integrator/2
  S-R Flip-Flop/2 -> Terminator/1
  Add/1 -> Ref/1
  Gain3/1 -> Add/1

== system PECommon/2BirdgePhaseShiftdriver/DutySampling ==
  In1 : Inport
  Trigger : TriggerPort
  Divide2 : Product  Inputs=**
  Saturation : Saturate  UpperLimit=1  LowerLimit=0
  Ts1 : Constant  Value=pi
  Ts2 : Constant  OutDataTypeStr=boolean
  LaggingTime : Outport
  LaggingEnable : Outport  Port=2  InitialOutput=[0]
  wires:
  Saturation/1 -> Divide2/1
  Ts1/1 -> Divide2/2
  In1/1 -> Saturation/1
  Divide2/1 -> LaggingTime/1
  Ts2/1 -> LaggingEnable/1

== system PECommon/Disturb/Custom ==
  Constant3 : Constant  Value=1e3
  Product : Product  RndMeth=Zero
  Repeating Sequence Stair : simulink/Sources/Repeating Sequence Stair  SystemSampleTime=-1  OutValues=Value.'  tsamp=TsCustom  OutMin=[]  OutMax=[]  OutDataTypeStr=double  OutputDataTypeScalingMode=double  OutDataType=fixdt(0,8)  ConRadixGroup=Best Precision: Vector-wise  OutScaling=2^-12
  Out1 : Outport
  wires:
  Repeating Sequence Stair/1 -> Product/1
  Product/1 -> Out1/1
  Constant3/1 -> Product/2

== system PECommon/Disturb/Pluse ==
  Add1 : Sum  Inputs=+-
  Add2 : Sum
  Constant1 : Constant  Value=(MaxP+MinP)/2
  Constant2 : Constant  Value=1e3
  Constant3 : Constant  Value=(MaxP-MinP)/2
  Product : Product  RndMeth=Zero
  Pulse Generator : DiscretePulseGenerator  PulseType=Time based  Amplitude=2e3  Period=PluseTs  PulseWidth=50
  Out1 : Outport
  wires:
  Pulse Generator/1 -> Add1/1
  Constant2/1 -> Add1/2
  Add1/1 -> Product/2
  Constant3/1 -> Product/1
  Product/1 -> Add2/1
  Add2/1 -> Out1/1
  Constant1/1 -> Add2/2

== system PECommon/Disturb/Step ==
  Step : Step  Time=StepT  Before=InitP*1e3  After=FinalP*1e3  SampleTime=0
  Out1 : Outport
  wires:
  Step/1 -> Out1/1
